simulink model "sim6"  (R2022a)
settings: Solver=FixedStepAuto  StartTime=0.0  StopTime=120  FixedStep=0.001  MaxStep=0.002  RelTol=1e-3
libraries: fl_lib x14, nesl_utility x7, dsparch4 x3, dspstat3 x2, dspadpt3 x1
settings Model: Creator=targi  LastModifiedBy=targi

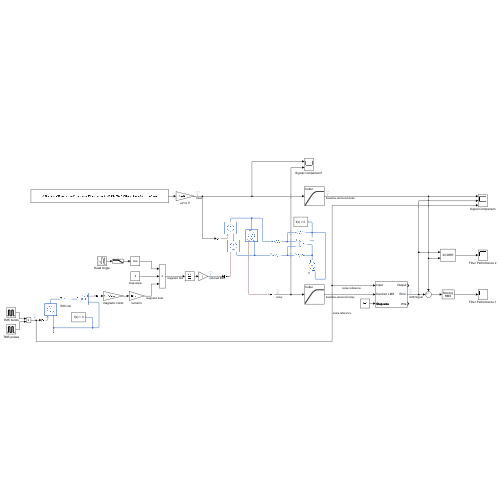
[thumbnail: Simulink's stored preview of the top-level diagram]
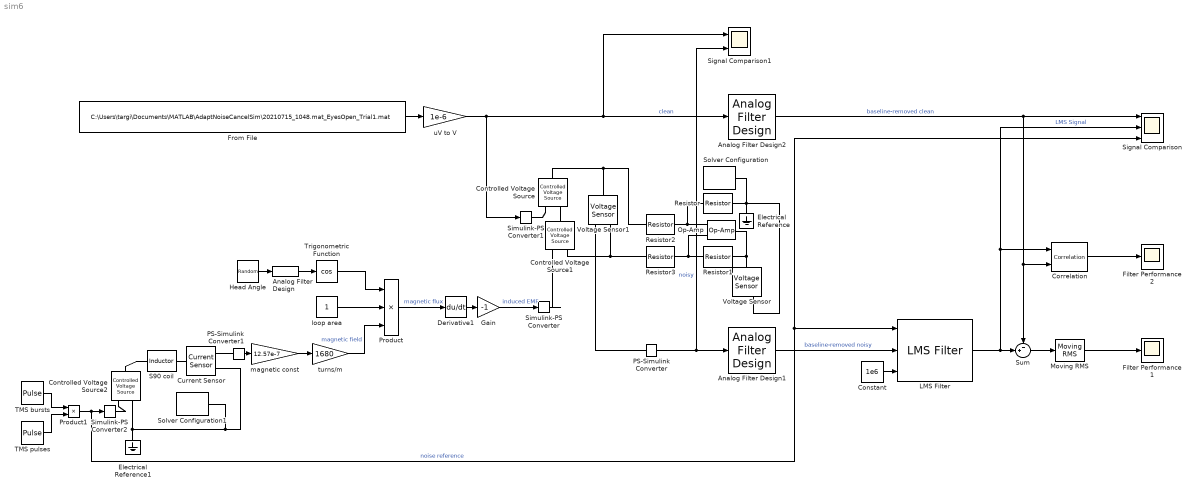
== system sim6 ==
  Analog Filter Design : dsparch4/Analog Filter Design  method=Butterworth  filttype=Lowpass  N=8  Wlo=100  Whi=80  Rp=2  Rs=40
  Analog Filter Design1 : dsparch4/Analog Filter Design  method=Butterworth  filttype=Highpass  N=2  Wlo=10  Whi=80  Rp=2  Rs=40
  Analog Filter Design2 : dsparch4/Analog Filter Design  method=Butterworth  filttype=Highpass  N=2  Wlo=10  Whi=80  Rp=2  Rs=40
  Constant : Constant  Value=1e6
  Controlled Voltage Source : fl_lib/Electrical/Electrical Sources/Controlled Voltage Source
      settings: SourceProductBaseCode=PW,SS,VE
  Controlled Voltage Source1 : fl_lib/Electrical/Electrical Sources/Controlled Voltage Source
      settings: SourceProductBaseCode=PW,SS,VE
  Controlled Voltage Source2 : fl_lib/Electrical/Electrical Sources/Controlled Voltage Source
      settings: SourceProductBaseCode=PW,SS,VE
  Correlation : dspstat3/Correlation  domain=Time  roundingMode=Floor  overflowMode=off  outputDataTypeStr=Inherit: Same as accumulator  outputMin=[]  outputMax=[]  outputLastDataTypeStr=Inherit: Same as accumulator
      settings: SourceProductBaseCode=DS
  Current Sensor : fl_lib/Electrical/Electrical Sensors/Current Sensor
      settings: SourceProductBaseCode=PW,SS,VE
  Derivative1 : Derivative
  Electrical Reference : fl_lib/Electrical/Electrical Elements/Electrical Reference
      settings: SourceProductBaseCode=PW,SS,VE
  Electrical Reference1 : fl_lib/Electrical/Electrical Elements/Electrical Reference
      settings: SourceProductBaseCode=PW,SS,VE
  Filter Performance 1 : Scope
  Filter Performance 2 : Scope
  From File : FromFile  FileName=C:\Users\targi\Documents\MATLAB\AdaptNoiseCancelSim\20210715_1048.mat_EyesOpen_Trial1.mat
  Gain : Gain  Gain=-1
  "Head Angle " : RandomNumber  Variance=.15
  LMS Filter : dspadpt3/LMS Filter  Algo=LMS  L=128  stepflag=Input port  mu=1e7  leakage=1  ic=0  Adapt=off  resetflag=None  weights=on  addnparflag=off  roundingMode=Floor  overflowMode=off  firstCoeffMode=Binary point scaling  firstCoeffWordLength=16  firstCoeffFracLength=15
      settings: SourceProductBaseCode=DS
  Moving RMS : dspstat3/Moving RMS  Method=Sliding window  ForgettingFactorPort=off  SpecifyWindowLength=on  WindowLength=5000  ForgettingFactor=0.9  SimulateUsing=Code generation
      settings: SourceProductBaseCode=DS
  Op-Amp : fl_lib/Electrical/Electrical Elements/Op-Amp  outI_specify=off  outI_priority=None  outI=0 A  outI_nominal_specify=off  outI_nominal_unit=A  outI_nominal_value=1
      settings: SourceProductBaseCode=PW,SS,VE
  PS-Simulink Converter : nesl_utility/PS-Simulink Converter  PhysicalDomain=network_engine_domain  SubClassName=ps_output  LeftPortType=input  RightPortType=output  PseudoPeriodic=off  Frequencies=[]  VectorFormat=inherit  Unit=inherit  AffineConversion=off
      settings: SourceProductBaseCode=SS,PW,VE
  PS-Simulink Converter1 : nesl_utility/PS-Simulink Converter  PhysicalDomain=network_engine_domain  SubClassName=ps_output  LeftPortType=input  RightPortType=output  PseudoPeriodic=off  Frequencies=[]  VectorFormat=inherit  Unit=inherit  AffineConversion=off
      settings: SourceProductBaseCode=SS,PW,VE
  Product : Product  Inputs=3
  Product1 : Product
  Resistor : fl_lib/Electrical/Electrical Elements/Resistor  R=100 Ohm  i_specify=off  i_priority=None  i=0 A  i_nominal_specify=off  i_nominal_unit=A  i_nominal_value=1  v_specify=off  v_priority=None  v=0 V  v_nominal_specify=off  v_nominal_unit=V  v_nominal_value=1
      settings: SourceProductBaseCode=PW,SS,VE
  Resistor1 : fl_lib/Electrical/Electrical Elements/Resistor  R=100 Ohm  i_specify=off  i_priority=None  i=0 A  i_nominal_specify=off  i_nominal_unit=A  i_nominal_value=1  v_specify=off  v_priority=None  v=0 V  v_nominal_specify=off  v_nominal_unit=V  v_nominal_value=1
      settings: SourceProductBaseCode=PW,SS,VE
  Resistor2 : fl_lib/Electrical/Electrical Elements/Resistor  R=1 Ohm  i_specify=off  i_priority=None  i=0 A  i_nominal_specify=off  i_nominal_unit=A  i_nominal_value=1  v_specify=off  v_priority=None  v=0 V  v_nominal_specify=off  v_nominal_unit=V  v_nominal_value=1
      settings: SourceProductBaseCode=PW,SS,VE
  Resistor3 : fl_lib/Electrical/Electrical Elements/Resistor  R=1 Ohm  i_specify=off  i_priority=None  i=0 A  i_nominal_specify=off  i_nominal_unit=A  i_nominal_value=1  v_specify=off  v_priority=None  v=0 V  v_nominal_specify=off  v_nominal_unit=V  v_nominal_value=1
      settings: SourceProductBaseCode=PW,SS,VE
  S90 coil : fl_lib/Electrical/Electrical Elements/Inductor  l=23.47 uH  r=.01 Ohm  g=1e-9 1/Ohm  i_specify=off  i_priority=None  i=0 A  i_nominal_specify=off  i_nominal_unit=A  i_nominal_value=1  v_specify=off  v_priority=None  v=0 V  v_nominal_specify=off  v_nominal_unit=V  v_nominal_value=1  i_L_specify=off  i_L_priority=High  i_L=0 A  i_L_nominal_specify=off  i_L_nominal_unit=A  i_L_nominal_value=1
      settings: SourceProductBaseCode=PW,SS,VE
  Signal Comparison : Scope  NumInputPorts=3
  Signal Comparison1 : Scope  NumInputPorts=2
  Simulink-PS Converter : nesl_utility/Simulink-PS Converter  PhysicalDomain=network_engine_domain  SubClassName=ps_input  LeftPortType=input  RightPortType=output  PseudoPeriodic=off  Frequencies=[]  NoiseDistribution=none  NoiseParameters=[]  Unit=1  AffineConversion=off  FilteringAndDerivatives=provide  SimscapeFilterOrder=1  InputFilterTimeConstant=0.001  UdotUserProvided=0
      settings: SourceProductBaseCode=SS,PW,VE
  Simulink-PS Converter1 : nesl_utility/Simulink-PS Converter  PhysicalDomain=network_engine_domain  SubClassName=ps_input  LeftPortType=input  RightPortType=output  PseudoPeriodic=off  Frequencies=[]  NoiseDistribution=none  NoiseParameters=[]  Unit=1  AffineConversion=off  FilteringAndDerivatives=provide  SimscapeFilterOrder=1  InputFilterTimeConstant=0.001  UdotUserProvided=0
      settings: SourceProductBaseCode=SS,PW,VE
  Simulink-PS Converter2 : nesl_utility/Simulink-PS Converter  PhysicalDomain=network_engine_domain  SubClassName=ps_input  LeftPortType=input  RightPortType=output  PseudoPeriodic=off  Frequencies=[]  NoiseDistribution=none  NoiseParameters=[]  Unit=1  AffineConversion=off  FilteringAndDerivatives=provide  SimscapeFilterOrder=1  InputFilterTimeConstant=0.001  UdotUserProvided=0
      settings: SourceProductBaseCode=SS,PW,VE
  Solver Configuration : nesl_utility/Solver Configuration  PhysicalDomain=network_engine_domain  SubClassName=solver  LeftPortType=input  RightPortType=generic  Tones=[]  Harmonics=[]  SimulateNoise=off  Profile=off  UseLocalSampling=off  EnableSwitchedLinearOptims=on  FrequencyDomain=off  UseCCode=off  RelTol=0.001  AbsTol=0.001  MinStep=1e-09  ToWorkspace=off  RevertToSquareIcSolve=off  NumHomotopyIterations=100  PhasorMode=off  PhasorModeNumHarmonics=1  IndexReductionMethod=DerivativeReplacement  DoDC=off  ResidualTolerance=1e-09  UseLocalSolver=off  LocalSolverChoice=NE_BACKWARD_EULER_ADVANCER  LocalSolverSampleTime=0.001  DoFixedCost=off  MaxNonlinIter=3  MaxModeIter=2  ComputeImpulses=off  ImpulseIterations=2  LinearAlgebra=auto  LinearAlgebraNumThread=0  EquationFormulation=NE_TIME_EF  DelaysMemoryBudget=1024  AutomaticFiltering=on  FilteringTimeConstant=0.001  PartitionStorageMethod=AS_NEEDED  PartitionMemoryBudget=1024  PartitionMethod=ROBUST
      settings: SourceProductBaseCode=SS,PW,VE
  Solver Configuration1 : nesl_utility/Solver Configuration  PhysicalDomain=network_engine_domain  SubClassName=solver  LeftPortType=input  RightPortType=generic  Tones=[]  Harmonics=[]  SimulateNoise=off  Profile=off  UseLocalSampling=off  EnableSwitchedLinearOptims=on  FrequencyDomain=off  UseCCode=off  RelTol=0.001  AbsTol=0.001  MinStep=1e-09  ToWorkspace=off  RevertToSquareIcSolve=off  NumHomotopyIterations=100  PhasorMode=off  PhasorModeNumHarmonics=1  IndexReductionMethod=DerivativeReplacement  DoDC=off  ResidualTolerance=1e-09  UseLocalSolver=off  LocalSolverChoice=NE_BACKWARD_EULER_ADVANCER  LocalSolverSampleTime=0.001  DoFixedCost=off  MaxNonlinIter=3  MaxModeIter=2  ComputeImpulses=off  ImpulseIterations=2  LinearAlgebra=auto  LinearAlgebraNumThread=0  EquationFormulation=NE_TIME_EF  DelaysMemoryBudget=1024  AutomaticFiltering=on  FilteringTimeConstant=0.001  PartitionStorageMethod=AS_NEEDED  PartitionMemoryBudget=1024  PartitionMethod=ROBUST
      settings: SourceProductBaseCode=SS,PW,VE
  Sum : Sum  Inputs=-+|
  TMS bursts : DiscretePulseGenerator  PulseType=Time based  Period=.02  PulseWidth=5
  TMS pulses : DiscretePulseGenerator  PulseType=Time based  Amplitude=1e-4  Period=.2  PulseWidth=29
  Trigonometric Function : Trigonometry  Operator=cos
  Voltage Sensor : fl_lib/Electrical/Electrical Sensors/Voltage Sensor
      settings: SourceProductBaseCode=PW,SS,VE
  Voltage Sensor1 : fl_lib/Electrical/Electrical Sensors/Voltage Sensor
      settings: SourceProductBaseCode=PW,SS,VE
  loop area : Constant
  magnetic const : Gain  Gain=12.57e-7
  turns/m : Gain  Gain=1680
  uV to V : Gain  Gain=1e-6
  wires:
  Product1/1 -> Simulink-PS Converter2/1, Signal Comparison/3, LMS Filter/1  "noise reference"
  uV to V/1 -> Signal Comparison1/1, Analog Filter Design2/1, Simulink-PS Converter1/1  "clean"
  PS-Simulink Converter/1 -> Signal Comparison1/2, Analog Filter Design1/1  "noisy"
  loop area/1 -> Product/2
  Trigonometric Function/1 -> Product/1
  Product/1 -> Derivative1/1  "magnetic flux"
  Derivative1/1 -> Gain/1
  Gain/1 -> Simulink-PS Converter/1  "induced EMF"
  "Head Angle "/1 -> Analog Filter Design/1
  Analog Filter Design/1 -> Trigonometric Function/1
  TMS bursts/1 -> Product1/1
  TMS pulses/1 -> Product1/2
  From File/1 -> uV to V/1
  PS-Simulink Converter1/1 -> magnetic const/1
  magnetic const/1 -> turns/m/1
  turns/m/1 -> Product/3  "magnetic field"
  Analog Filter Design1/1 -> LMS Filter/2  "baseline-removed noisy"
  Constant/1 -> LMS Filter/3
  Analog Filter Design2/1 -> Signal Comparison/1, Correlation/2, Sum/1  "baseline-removed clean"
  LMS Filter/2 -> Sum/2, Signal Comparison/2, Correlation/1  "LMS Signal"
  Sum/1 -> Moving RMS/1
  Moving RMS/1 -> Filter Performance 1/1
  Correlation/1 -> Filter Performance 2/1
  connections:
  Resistor2/RConn1 -- Op-Amp/LConn1 -- Resistor/LConn1
  Resistor1/LConn1 -- Op-Amp/LConn2 -- Resistor3/RConn1
  Op-Amp/RConn1 -- Resistor1/RConn1 -- Voltage Sensor/LConn1
  Resistor/RConn1 -- Solver Configuration/RConn1 -- Electrical Reference/LConn1 -- Voltage Sensor/RConn2
  Resistor2/LConn1 -- Controlled Voltage Source/LConn1 -- Voltage Sensor1/LConn1
  Controlled Voltage Source1/LConn1 -- Controlled Voltage Source/RConn2
  Voltage Sensor1/RConn2 -- Controlled Voltage Source1/RConn2 -- Resistor3/LConn1
  Simulink-PS Converter/RConn1 -- Controlled Voltage Source1/RConn1
  Simulink-PS Converter1/RConn1 -- Controlled Voltage Source/RConn1
  Voltage Sensor1/RConn1 -- PS-Simulink Converter/LConn1
  Simulink-PS Converter2/RConn1 -- Controlled Voltage Source2/RConn1
  S90 coil/LConn1 -- Controlled Voltage Source2/LConn1
  S90 coil/RConn1 -- Current Sensor/LConn1
  Current Sensor/RConn2 -- Controlled Voltage Source2/RConn2 -- Electrical Reference1/LConn1 -- Solver Configuration1/RConn1
  PS-Simulink Converter1/LConn1 -- Current Sensor/RConn1
